simulink model "siulin_atempt - Copy"  (R2023a)
settings: Solver=VariableStepAuto  StartTime=0.0  StopTime=100  RelTol=1e-3
undefined symbols (not defined in the file or in its folder): k_ave
settings Model: Creator=kianf  LastModifiedBy=kianf

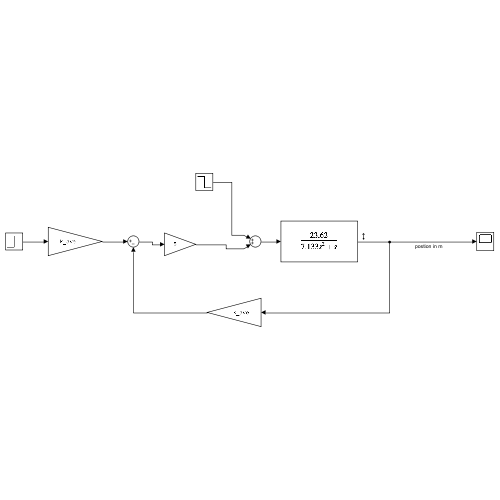
[thumbnail: Simulink's stored preview of the top-level diagram]
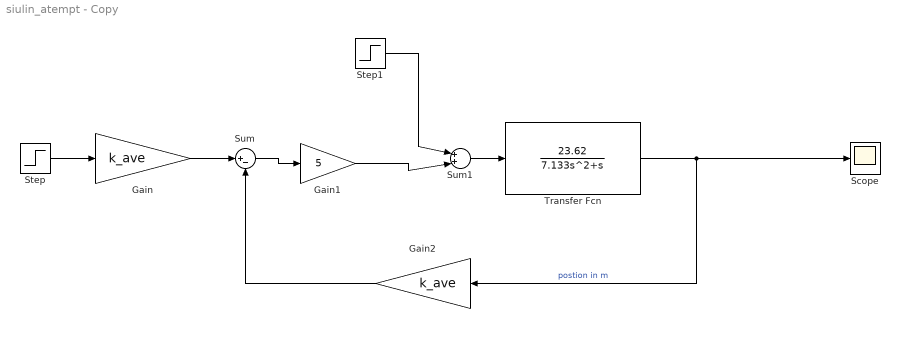
== system siulin_atempt - Copy ==
  Gain : Gain  Gain=k_ave
  Gain1 : Gain  Gain=5
  Gain2 : Gain  Gain=k_ave
  Scope : Scope
  Step : Step  SampleTime=0
  Step1 : Step  After=-2.5  SampleTime=0
  Sum : Sum  Inputs=|+-
  Sum1 : Sum  Inputs=|++|
  Transfer Fcn : TransferFcn  Numerator=[23.62]  Denominator=[7.133 1 0]
  wires:
  Step/1 -> Gain/1
  Gain/1 -> Sum/1
  Gain1/1 -> Sum1/2
  Sum1/1 -> Transfer Fcn/1
  Transfer Fcn/1 -> Gain2/1, Scope/1  "postion in m"
  Sum/1 -> Gain1/1
  Step1/1 -> Sum1/1
  Gain2/1 -> Sum/2
